simulink model "ikine_test"  (R2019b)
settings: Solver=ode45  StartTime=0.0  StopTime=10.0  RelTol=1e-3  EnableMultiTasking=on
values from neighbouring files (symbols this model uses):
  bL = 22    [runfirst.m]
  bWb = 15.5    [runfirst.m]
  bWs = 13.5    [runfirst.m]
  d1 = 0    [runfirst.m]
  d2 = 0    [runfirst.m]
  L1 = 3.4    [runfirst.m]
  L2 = 9.5    [runfirst.m]
  L3 = 14.2    [runfirst.m]
settings Model: Creator=340DANILOV  LastModifiedBy=root
settings DataIOCC: LimitDataPoints=on  SaveFormat=Array  ReturnWorkspaceOutputs=off
settings OptimizationCC: LifeSpan=inf
settings DebuggingCC: SFUnexpectedBacktrackingDiag=warning  SFNoUnconditionalDefaultTransitionDiag=warning  SFExecutionAtInitializationDiag=none  UnderSpecifiedDimensionMsg=warning  ArithmeticOperatorsInVariantConditions=warning
settings HardwareCC: ProdBitPerPointer=32  ProdBitPerSizeT=32  ProdBitPerPtrDiffT=32  ProdLargestAtomicFloat=None  ProdIntDivRoundTo=Undefined  ProdEndianess=Unspecified  ProdWordSize=32  ProdHWDeviceType=32-bit Generic
settings ModelReferenceCC: PropagateSignalLabelsOutOfModel=off
settings SFSimCC: SimUseLocalCustomCode=off  CustomCodeUndefinedFunction=UseInterfaceOnly
settings RTWCC: RTWUseLocalCustomCode=off
settings CodeAppCC: StateflowObjectComments=on
settings GRTTargetCC: TargetLangStandard=C89/C90 (ANSI)  GeneratePreprocessorConditionals=Disable all
settings ConfigComp: CovMetricSettings=dw  CovHtmlReporting=on  CovSaveCumulativeToWorkspaceVar=on  CovSaveSingleToWorkspaceVar=on  CovExternalEMLEnable=off

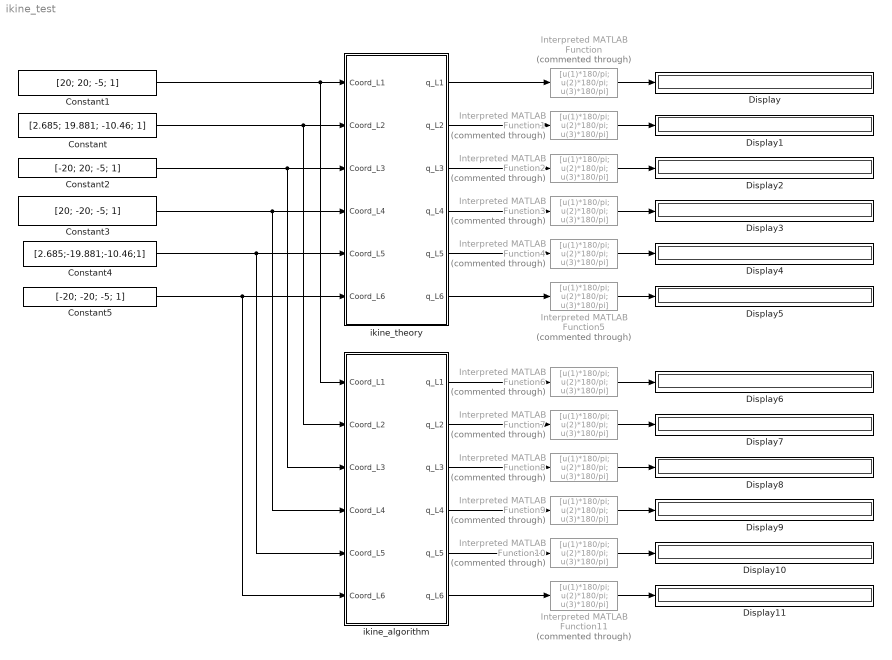
== system ikine_test ==
  Constant : Constant  Value=[2.685; 19.881; -10.46; 1]  VectorParams1D=off
  Constant1 : Constant  Value=[20; 20; -5; 1]  VectorParams1D=off
  Constant2 : Constant  Value=[-20; 20; -5; 1]  VectorParams1D=off
  Constant3 : Constant  Value=[20; -20; -5; 1]  VectorParams1D=off
  Constant4 : Constant  Value=[2.685;-19.881;-10.46;1]  VectorParams1D=off
  Constant5 : Constant  Value=[-20; -20; -5; 1]  VectorParams1D=off
  Display{,1..11} (12 alike) : Display
  Interpreted MATLAB Function{,1..11} (12 alike) : MATLABFcn  Commented=through  MATLABFcn=[u(1)*180/pi; u(2)*180/pi; u(3)*180/pi]
  ikine_algorithm : Subsystem
  ikine_theory : Subsystem
  wires:
  Constant/1 -> ikine_algorithm/2(Coord_L2), ikine_theory/2(Coord_L2)
  Constant1/1 -> ikine_algorithm/1(Coord_L1), ikine_theory/1(Coord_L1)
  Constant2/1 -> ikine_algorithm/3(Coord_L3), ikine_theory/3(Coord_L3)
  Constant3/1 -> ikine_algorithm/4(Coord_L4), ikine_theory/4(Coord_L4)
  Constant4/1 -> ikine_algorithm/5(Coord_L5), ikine_theory/5(Coord_L5)
  Constant5/1 -> ikine_algorithm/6(Coord_L6), ikine_theory/6(Coord_L6)
  Interpreted MATLAB Function/1 -> Display/1
  ikine_theory/1(q_L1) -> Interpreted MATLAB Function/1
  ikine_theory/2(q_L2) -> Interpreted MATLAB Function1/1
  Interpreted MATLAB Function1/1 -> Display1/1
  ikine_theory/3(q_L3) -> Interpreted MATLAB Function2/1
  Interpreted MATLAB Function2/1 -> Display2/1
  ikine_theory/4(q_L4) -> Interpreted MATLAB Function3/1
  Interpreted MATLAB Function3/1 -> Display3/1
  ikine_theory/5(q_L5) -> Interpreted MATLAB Function4/1
  Interpreted MATLAB Function4/1 -> Display4/1
  ikine_theory/6(q_L6) -> Interpreted MATLAB Function5/1
  Interpreted MATLAB Function5/1 -> Display5/1
  ikine_algorithm/1(q_L1) -> Interpreted MATLAB Function6/1
  Interpreted MATLAB Function6/1 -> Display6/1
  ikine_algorithm/2(q_L2) -> Interpreted MATLAB Function7/1
  Interpreted MATLAB Function7/1 -> Display7/1
  ikine_algorithm/3(q_L3) -> Interpreted MATLAB Function8/1
  Interpreted MATLAB Function8/1 -> Display8/1
  ikine_algorithm/4(q_L4) -> Interpreted MATLAB Function9/1
  Interpreted MATLAB Function9/1 -> Display9/1
  ikine_algorithm/5(q_L5) -> Interpreted MATLAB Function10/1
  Interpreted MATLAB Function10/1 -> Display10/1
  ikine_algorithm/6(q_L6) -> Interpreted MATLAB Function11/1
  Interpreted MATLAB Function11/1 -> Display11/1

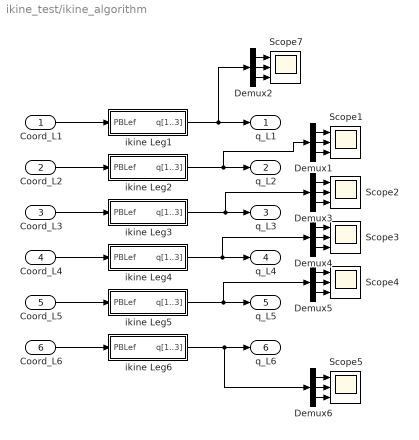
== system ikine_test/ikine_algorithm ==
  Coord_L1 : Inport
  Coord_L2 : Inport  Port=2
  Coord_L3 : Inport  Port=3
  Coord_L4 : Inport  Port=4
  Coord_L5 : Inport  Port=5
  Coord_L6 : Inport  Port=6
  Demux{1..6} (6 alike) : Demux  Outputs=3
  Scope{1..5,7} (6 alike) : Scope  NumInputPorts=3
  ikine Leg1 : Subsystem
  ikine Leg2 : Subsystem
  ikine Leg3 : Subsystem
  ikine Leg4 : Subsystem
  ikine Leg5 : Subsystem
  ikine Leg6 : Subsystem
  q_L1 : Outport  VectorParamsAs1DForOutWhenUnconnected=off
  q_L2 : Outport  Port=2  VectorParamsAs1DForOutWhenUnconnected=off
  q_L3 : Outport  Port=3  VectorParamsAs1DForOutWhenUnconnected=off
  q_L4 : Outport  Port=4  VectorParamsAs1DForOutWhenUnconnected=off
  q_L5 : Outport  Port=5  VectorParamsAs1DForOutWhenUnconnected=off
  q_L6 : Outport  Port=6  VectorParamsAs1DForOutWhenUnconnected=off
  wires:
  Demux6/1 -> Scope5/1
  Demux6/2 -> Scope5/2
  Demux6/3 -> Scope5/3
  Demux5/1 -> Scope4/1
  Demux5/2 -> Scope4/2
  Demux5/3 -> Scope4/3
  Demux4/1 -> Scope3/1
  Demux4/2 -> Scope3/2
  Demux4/3 -> Scope3/3
  Demux3/1 -> Scope2/1
  Demux3/2 -> Scope2/2
  Demux3/3 -> Scope2/3
  Demux1/1 -> Scope1/1
  Demux1/2 -> Scope1/2
  Demux1/3 -> Scope1/3
  Demux2/1 -> Scope7/1
  Demux2/2 -> Scope7/2
  Demux2/3 -> Scope7/3
  Coord_L6/1 -> ikine Leg6/1(PBLef)
  Coord_L5/1 -> ikine Leg5/1(PBLef)
  Coord_L4/1 -> ikine Leg4/1(PBLef)
  Coord_L3/1 -> ikine Leg3/1(PBLef)
  Coord_L2/1 -> ikine Leg2/1(PBLef)
  Coord_L1/1 -> ikine Leg1/1(PBLef)
  ikine Leg6/1(q[1..3]) -> q_L6/1, Demux6/1
  ikine Leg5/1(q[1..3]) -> q_L5/1, Demux5/1
  ikine Leg4/1(q[1..3]) -> q_L4/1, Demux4/1
  ikine Leg3/1(q[1..3]) -> q_L3/1, Demux3/1
  ikine Leg2/1(q[1..3]) -> q_L2/1, Demux1/1
  ikine Leg1/1(q[1..3]) -> q_L1/1, Demux2/1

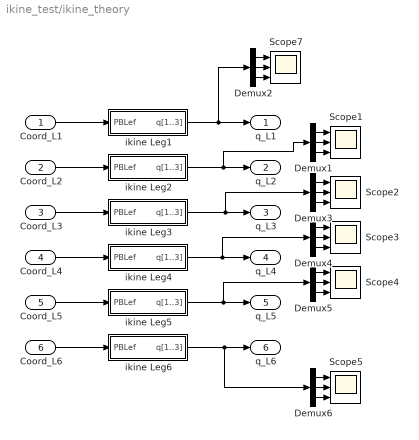
== system ikine_test/ikine_theory ==
  Coord_L1 : Inport
  Coord_L2 : Inport  Port=2
  Coord_L3 : Inport  Port=3
  Coord_L4 : Inport  Port=4
  Coord_L5 : Inport  Port=5
  Coord_L6 : Inport  Port=6
  Demux{1..6} (6 alike) : Demux  Outputs=3
  Scope{1..5,7} (6 alike) : Scope  NumInputPorts=3
  ikine Leg1 : Subsystem
  ikine Leg2 : Subsystem
  ikine Leg3 : Subsystem
  ikine Leg4 : Subsystem
  ikine Leg5 : Subsystem
  ikine Leg6 : Subsystem
  q_L1 : Outport  VectorParamsAs1DForOutWhenUnconnected=off
  q_L2 : Outport  Port=2  VectorParamsAs1DForOutWhenUnconnected=off
  q_L3 : Outport  Port=3  VectorParamsAs1DForOutWhenUnconnected=off
  q_L4 : Outport  Port=4  VectorParamsAs1DForOutWhenUnconnected=off
  q_L5 : Outport  Port=5  VectorParamsAs1DForOutWhenUnconnected=off
  q_L6 : Outport  Port=6  VectorParamsAs1DForOutWhenUnconnected=off
  wires:
  Demux6/1 -> Scope5/1
  Demux6/2 -> Scope5/2
  Demux6/3 -> Scope5/3
  Demux5/1 -> Scope4/1
  Demux5/2 -> Scope4/2
  Demux5/3 -> Scope4/3
  Demux4/1 -> Scope3/1
  Demux4/2 -> Scope3/2
  Demux4/3 -> Scope3/3
  Demux3/1 -> Scope2/1
  Demux3/2 -> Scope2/2
  Demux3/3 -> Scope2/3
  Demux1/1 -> Scope1/1
  Demux1/2 -> Scope1/2
  Demux1/3 -> Scope1/3
  Demux2/1 -> Scope7/1
  Demux2/2 -> Scope7/2
  Demux2/3 -> Scope7/3
  Coord_L6/1 -> ikine Leg6/1(PBLef)
  Coord_L5/1 -> ikine Leg5/1(PBLef)
  Coord_L4/1 -> ikine Leg4/1(PBLef)
  Coord_L3/1 -> ikine Leg3/1(PBLef)
  Coord_L2/1 -> ikine Leg2/1(PBLef)
  Coord_L1/1 -> ikine Leg1/1(PBLef)
  ikine Leg6/1(q[1..3]) -> q_L6/1, Demux6/1
  ikine Leg5/1(q[1..3]) -> q_L5/1, Demux5/1
  ikine Leg4/1(q[1..3]) -> q_L4/1, Demux4/1
  ikine Leg3/1(q[1..3]) -> q_L3/1, Demux3/1
  ikine Leg2/1(q[1..3]) -> q_L2/1, Demux1/1
  ikine Leg1/1(q[1..3]) -> q_L1/1, Demux2/1

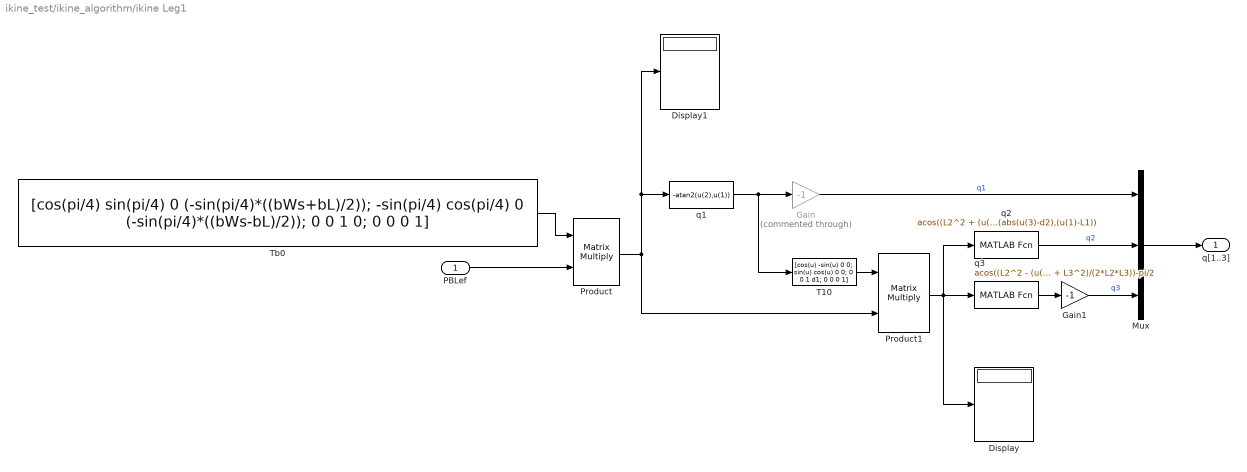
== system ikine_test/ikine_algorithm/ikine Leg1 ==
  PBLef : Inport
  Display : Display
  Display1 : Display
  Gain : Gain  Commented=through  Gain=-1
  Gain1 : Gain  Gain=-1
  Mux : Mux  Inputs=3
  Product : Product  Multiplication=Matrix(*)
  Product1 : Product  Multiplication=Matrix(*)
  T10 : MATLABFcn  MATLABFcn=[cos(u) -sin(u) 0 0; sin(u) cos(u) 0 0; 0 0 1 d1; 0 0 0 1]  OutputDimensions=[4;4]  Output1D=off
  Tb0 : Constant  Value=[cos(pi/4) sin(pi/4) 0 (-sin(pi/4)*((bWs+bL)/2)); -sin(pi/4) cos(pi/4) 0 (-sin(pi/4)*((bWs-bL)/2)); 0 0 1 0; 0 0 0 1]  VectorParams1D=off
  q1 : MATLABFcn  MATLABFcn=-atan2(u(2),u(1))
  q2 : MATLABFcn  MATLABFcn=acos((L2^2 + (u(1)-L1)^2 + (u(3)-d2)^2 - L3^2)/(2*L2*sqrt((u(1)-L1)^2+(u(3)-d2)^2)))-atan2(abs(u(3)-d2),(u(1)-L1))
  q3 : MATLABFcn  MATLABFcn=acos((L2^2 - (u(1)-L1)^2 - (u(3)-d2)^2 + L3^2)/(2*L2*L3))-pi/2
  q[1..3] : Outport  VectorParamsAs1DForOutWhenUnconnected=off
  wires:
  Gain1/1 -> Mux/3  "q3"
  Tb0/1 -> Product/1
  PBLef/1 -> Product/2
  Product/1 -> Display1/1, q1/1, Product1/2
  q1/1 -> T10/1, Gain/1
  q2/1 -> Mux/2  "q2"
  T10/1 -> Product1/1
  Product1/1 -> Display/1, q3/1, q2/1
  q3/1 -> Gain1/1
  Gain/1 -> Mux/1  "q1"
  Mux/1 -> q[1..3]/1

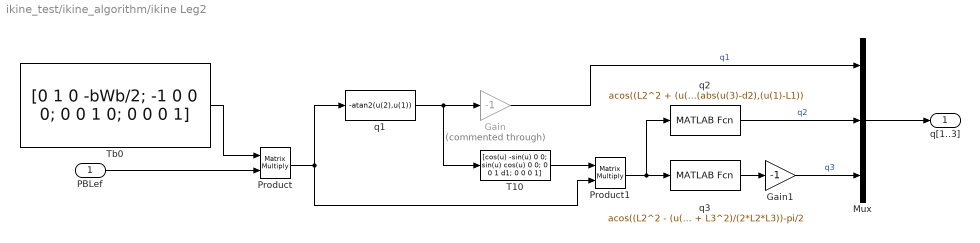
== system ikine_test/ikine_algorithm/ikine Leg2 ==
  PBLef : Inport
  Gain : Gain  Commented=through  Gain=-1
  Gain1 : Gain  Gain=-1
  Mux : Mux  Inputs=3
  Product : Product  Multiplication=Matrix(*)
  Product1 : Product  Multiplication=Matrix(*)
  T10 : MATLABFcn  MATLABFcn=[cos(u) -sin(u) 0 0; sin(u) cos(u) 0 0; 0 0 1 d1; 0 0 0 1]  OutputDimensions=[4;4]  Output1D=off
  Tb0 : Constant  Value=[0 1 0 -bWb/2; -1 0 0 0; 0 0 1 0; 0 0 0 1]  VectorParams1D=off
  q1 : MATLABFcn  MATLABFcn=-atan2(u(2),u(1))
  q2 : MATLABFcn  MATLABFcn=acos((L2^2 + (u(1)-L1)^2 + (u(3)-d2)^2 - L3^2)/(2*L2*sqrt((u(1)-L1)^2+(u(3)-d2)^2)))-atan2(abs(u(3)-d2),(u(1)-L1))
  q3 : MATLABFcn  MATLABFcn=acos((L2^2 - (u(1)-L1)^2 - (u(3)-d2)^2 + L3^2)/(2*L2*L3))-pi/2
  q[1..3] : Outport  VectorParamsAs1DForOutWhenUnconnected=off
  wires:
  Gain1/1 -> Mux/3  "q3"
  Tb0/1 -> Product/1
  PBLef/1 -> Product/2
  Product/1 -> q1/1, Product1/2
  q1/1 -> T10/1, Gain/1
  q2/1 -> Mux/2  "q2"
  T10/1 -> Product1/1
  Product1/1 -> q3/1, q2/1
  q3/1 -> Gain1/1
  Gain/1 -> Mux/1  "q1"
  Mux/1 -> q[1..3]/1

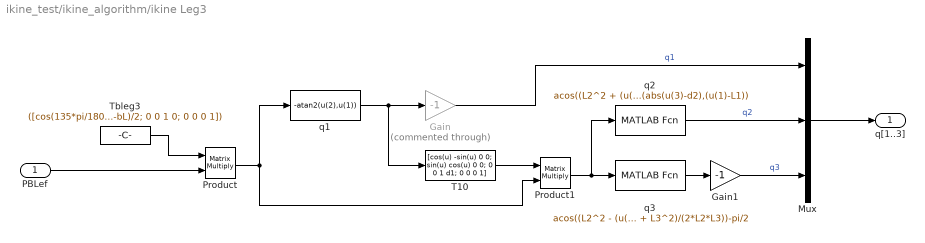
== system ikine_test/ikine_algorithm/ikine Leg3 ==
  PBLef : Inport
  Gain : Gain  Commented=through  Gain=-1
  Gain1 : Gain  Gain=-1
  Mux : Mux  Inputs=3
  Product : Product  Multiplication=Matrix(*)
  Product1 : Product  Multiplication=Matrix(*)
  T10 : MATLABFcn  MATLABFcn=[cos(u) -sin(u) 0 0; sin(u) cos(u) 0 0; 0 0 1 d1; 0 0 0 1]  OutputDimensions=[4;4]  Output1D=off
  Tbleg3 : Constant  Value=([cos(135*pi/180) sin(135*pi/180) 0 -sin(pi/4)*(bWs+bL)/2; sin(-135*pi/180) cos(135*pi/180) 0 sin(pi/4)*(bWs-bL)/2; 0 0 1 0; 0 0 0 1])  VectorParams1D=off
  q1 : MATLABFcn  MATLABFcn=-atan2(u(2),u(1))
  q2 : MATLABFcn  MATLABFcn=acos((L2^2 + (u(1)-L1)^2 + (u(3)-d2)^2 - L3^2)/(2*L2*sqrt((u(1)-L1)^2+(u(3)-d2)^2)))-atan2(abs(u(3)-d2),(u(1)-L1))
  q3 : MATLABFcn  MATLABFcn=acos((L2^2 - (u(1)-L1)^2 - (u(3)-d2)^2 + L3^2)/(2*L2*L3))-pi/2
  q[1..3] : Outport  VectorParamsAs1DForOutWhenUnconnected=off
  wires:
  Mux/1 -> q[1..3]/1
  Gain/1 -> Mux/1  "q1"
  q3/1 -> Gain1/1
  Product1/1 -> q2/1, q3/1
  T10/1 -> Product1/1
  q2/1 -> Mux/2  "q2"
  q1/1 -> T10/1, Gain/1
  Product/1 -> Product1/2, q1/1
  PBLef/1 -> Product/2
  Tbleg3/1 -> Product/1
  Gain1/1 -> Mux/3  "q3"

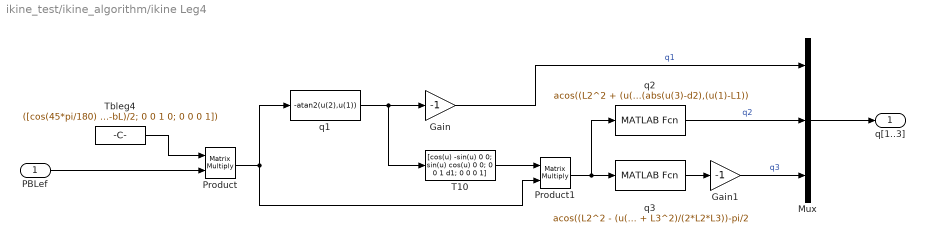
== system ikine_test/ikine_algorithm/ikine Leg4 ==
  PBLef : Inport
  Gain : Gain  Gain=-1
  Gain1 : Gain  Gain=-1
  Mux : Mux  Inputs=3
  Product : Product  Multiplication=Matrix(*)
  Product1 : Product  Multiplication=Matrix(*)
  T10 : MATLABFcn  MATLABFcn=[cos(u) -sin(u) 0 0; sin(u) cos(u) 0 0; 0 0 1 d1; 0 0 0 1]  OutputDimensions=[4;4]  Output1D=off
  Tbleg4 : Constant  Value=([cos(45*pi/180) -sin(45*pi/180) 0 -sin(pi/4)*(bWs+bL)/2; sin(45*pi/180) cos(45*pi/180) 0 sin(pi/4)*(bWs-bL)/2; 0 0 1 0; 0 0 0 1])  VectorParams1D=off
  q1 : MATLABFcn  MATLABFcn=-atan2(u(2),u(1))
  q2 : MATLABFcn  MATLABFcn=acos((L2^2 + (u(1)-L1)^2 + (u(3)-d2)^2 - L3^2)/(2*L2*sqrt((u(1)-L1)^2+(u(3)-d2)^2)))-atan2(abs(u(3)-d2),(u(1)-L1))
  q3 : MATLABFcn  MATLABFcn=acos((L2^2 - (u(1)-L1)^2 - (u(3)-d2)^2 + L3^2)/(2*L2*L3))-pi/2
  q[1..3] : Outport  VectorParamsAs1DForOutWhenUnconnected=off
  wires:
  Gain1/1 -> Mux/3  "q3"
  Tbleg4/1 -> Product/1
  PBLef/1 -> Product/2
  Product/1 -> q1/1, Product1/2
  q1/1 -> T10/1, Gain/1
  q2/1 -> Mux/2  "q2"
  T10/1 -> Product1/1
  Product1/1 -> q3/1, q2/1
  q3/1 -> Gain1/1
  Gain/1 -> Mux/1  "q1"
  Mux/1 -> q[1..3]/1

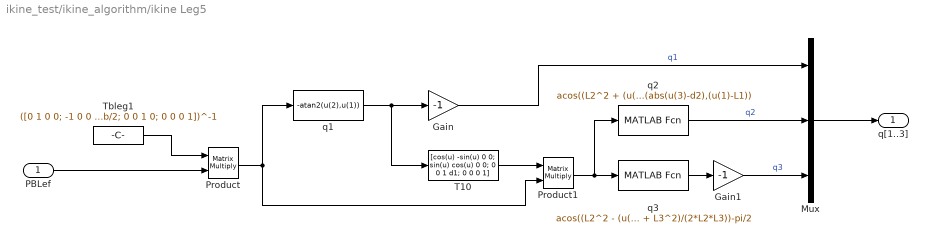
== system ikine_test/ikine_algorithm/ikine Leg5 ==
  PBLef : Inport
  Gain : Gain  Gain=-1
  Gain1 : Gain  Gain=-1
  Mux : Mux  Inputs=3
  Product : Product  Multiplication=Matrix(*)
  Product1 : Product  Multiplication=Matrix(*)
  T10 : MATLABFcn  MATLABFcn=[cos(u) -sin(u) 0 0; sin(u) cos(u) 0 0; 0 0 1 d1; 0 0 0 1]  OutputDimensions=[4;4]  Output1D=off
  Tbleg1 : Constant  Value=([0 1 0 0; -1 0 0 -bWb/2; 0 0 1 0; 0 0 0 1])^-1  VectorParams1D=off
  q1 : MATLABFcn  MATLABFcn=-atan2(u(2),u(1))
  q2 : MATLABFcn  MATLABFcn=acos((L2^2 + (u(1)-L1)^2 + (u(3)-d2)^2 - L3^2)/(2*L2*sqrt((u(1)-L1)^2+(u(3)-d2)^2)))-atan2(abs(u(3)-d2),(u(1)-L1))
  q3 : MATLABFcn  MATLABFcn=acos((L2^2 - (u(1)-L1)^2 - (u(3)-d2)^2 + L3^2)/(2*L2*L3))-pi/2
  q[1..3] : Outport  VectorParamsAs1DForOutWhenUnconnected=off
  wires:
  Mux/1 -> q[1..3]/1
  Gain/1 -> Mux/1  "q1"
  q3/1 -> Gain1/1
  Product1/1 -> q2/1, q3/1
  T10/1 -> Product1/1
  q2/1 -> Mux/2  "q2"
  q1/1 -> T10/1, Gain/1
  Product/1 -> Product1/2, q1/1
  PBLef/1 -> Product/2
  Tbleg1/1 -> Product/1
  Gain1/1 -> Mux/3  "q3"

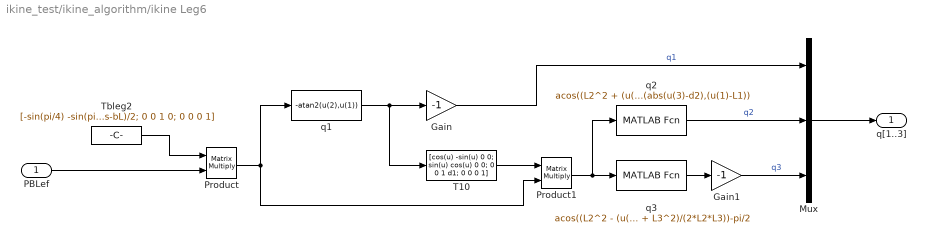
== system ikine_test/ikine_algorithm/ikine Leg6 ==
  PBLef : Inport
  Gain : Gain  Gain=-1
  Gain1 : Gain  Gain=-1
  Mux : Mux  Inputs=3
  Product : Product  Multiplication=Matrix(*)
  Product1 : Product  Multiplication=Matrix(*)
  T10 : MATLABFcn  MATLABFcn=[cos(u) -sin(u) 0 0; sin(u) cos(u) 0 0; 0 0 1 d1; 0 0 0 1]  OutputDimensions=[4;4]  Output1D=off
  Tbleg2 : Constant  Value=[-sin(pi/4) -sin(pi/4) 0 -sin(pi/4)*(bWs+bL)/2; sin(pi/4) -sin(pi/4) 0 -sin(pi/4)*(bWs-bL)/2; 0 0 1 0; 0 0 0 1]  VectorParams1D=off
  q1 : MATLABFcn  MATLABFcn=-atan2(u(2),u(1))
  q2 : MATLABFcn  MATLABFcn=acos((L2^2 + (u(1)-L1)^2 + (u(3)-d2)^2 - L3^2)/(2*L2*sqrt((u(1)-L1)^2+(u(3)-d2)^2)))-atan2(abs(u(3)-d2),(u(1)-L1))
  q3 : MATLABFcn  MATLABFcn=acos((L2^2 - (u(1)-L1)^2 - (u(3)-d2)^2 + L3^2)/(2*L2*L3))-pi/2
  q[1..3] : Outport  VectorParamsAs1DForOutWhenUnconnected=off
  wires:
  Mux/1 -> q[1..3]/1
  Gain/1 -> Mux/1  "q1"
  q3/1 -> Gain1/1
  Product1/1 -> q2/1, q3/1
  T10/1 -> Product1/1
  q2/1 -> Mux/2  "q2"
  q1/1 -> T10/1, Gain/1
  Product/1 -> Product1/2, q1/1
  PBLef/1 -> Product/2
  Tbleg2/1 -> Product/1
  Gain1/1 -> Mux/3  "q3"

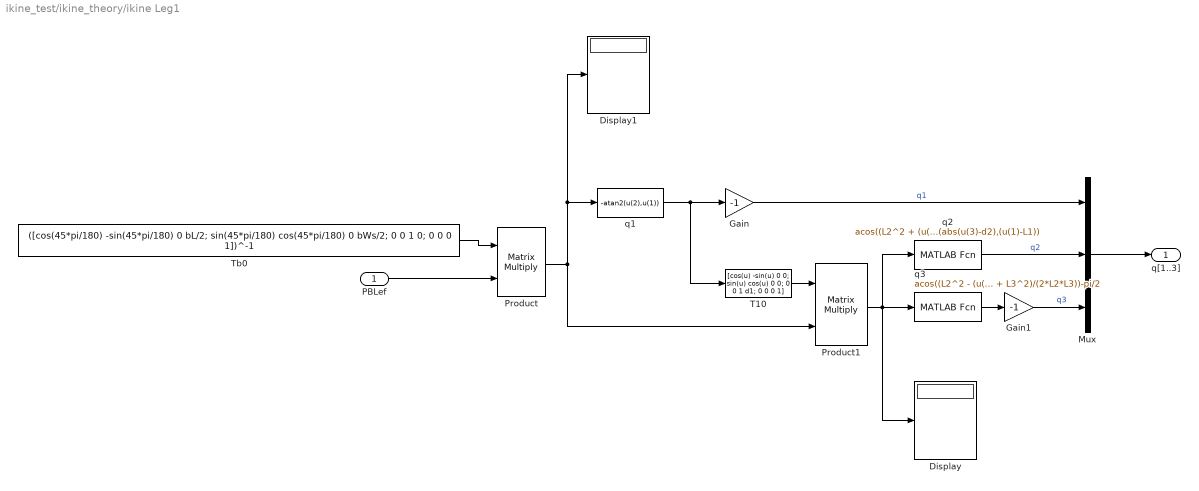
== system ikine_test/ikine_theory/ikine Leg1 ==
  PBLef : Inport
  Display : Display
  Display1 : Display
  Gain : Gain  Gain=-1
  Gain1 : Gain  Gain=-1
  Mux : Mux  Inputs=3
  Product : Product  Multiplication=Matrix(*)
  Product1 : Product  Multiplication=Matrix(*)
  T10 : MATLABFcn  MATLABFcn=[cos(u) -sin(u) 0 0; sin(u) cos(u) 0 0; 0 0 1 d1; 0 0 0 1]  Output1D=off
  Tb0 : Constant  Value=([cos(45*pi/180) -sin(45*pi/180) 0 bL/2; sin(45*pi/180) cos(45*pi/180) 0 bWs/2; 0 0 1 0; 0 0 0 1])^-1  VectorParams1D=off
  q1 : MATLABFcn  MATLABFcn=-atan2(u(2),u(1))
  q2 : MATLABFcn  MATLABFcn=acos((L2^2 + (u(1)-L1)^2 + (u(3)-d2)^2 - L3^2)/(2*L2*sqrt((u(1)-L1)^2+(u(3)-d2)^2)))-atan2(abs(u(3)-d2),(u(1)-L1))
  q3 : MATLABFcn  MATLABFcn=acos((L2^2 - (u(1)-L1)^2 - (u(3)-d2)^2 + L3^2)/(2*L2*L3))-pi/2
  q[1..3] : Outport  VectorParamsAs1DForOutWhenUnconnected=off
  wires:
  Gain1/1 -> Mux/3  "q3"
  Tb0/1 -> Product/1
  PBLef/1 -> Product/2
  Product/1 -> Display1/1, q1/1, Product1/2
  q1/1 -> T10/1, Gain/1
  q2/1 -> Mux/2  "q2"
  T10/1 -> Product1/1
  Product1/1 -> Display/1, q3/1, q2/1
  q3/1 -> Gain1/1
  Gain/1 -> Mux/1  "q1"
  Mux/1 -> q[1..3]/1

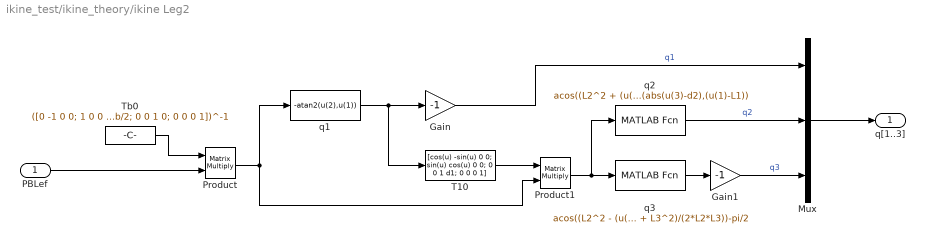
== system ikine_test/ikine_theory/ikine Leg2 ==
  PBLef : Inport
  Gain : Gain  Gain=-1
  Gain1 : Gain  Gain=-1
  Mux : Mux  Inputs=3
  Product : Product  Multiplication=Matrix(*)
  Product1 : Product  Multiplication=Matrix(*)
  T10 : MATLABFcn  MATLABFcn=[cos(u) -sin(u) 0 0; sin(u) cos(u) 0 0; 0 0 1 d1; 0 0 0 1]  OutputDimensions=[4;4]  Output1D=off
  Tb0 : Constant  Value=([0 -1 0 0; 1 0 0 bWb/2; 0 0 1 0; 0 0 0 1])^-1  VectorParams1D=off
  q1 : MATLABFcn  MATLABFcn=-atan2(u(2),u(1))
  q2 : MATLABFcn  MATLABFcn=acos((L2^2 + (u(1)-L1)^2 + (u(3)-d2)^2 - L3^2)/(2*L2*sqrt((u(1)-L1)^2+(u(3)-d2)^2)))-atan2(abs(u(3)-d2),(u(1)-L1))
  q3 : MATLABFcn  MATLABFcn=acos((L2^2 - (u(1)-L1)^2 - (u(3)-d2)^2 + L3^2)/(2*L2*L3))-pi/2
  q[1..3] : Outport  VectorParamsAs1DForOutWhenUnconnected=off
  wires:
  Gain1/1 -> Mux/3  "q3"
  Tb0/1 -> Product/1
  PBLef/1 -> Product/2
  Product/1 -> q1/1, Product1/2
  q1/1 -> T10/1, Gain/1
  q2/1 -> Mux/2  "q2"
  T10/1 -> Product1/1
  Product1/1 -> q3/1, q2/1
  q3/1 -> Gain1/1
  Gain/1 -> Mux/1  "q1"
  Mux/1 -> q[1..3]/1

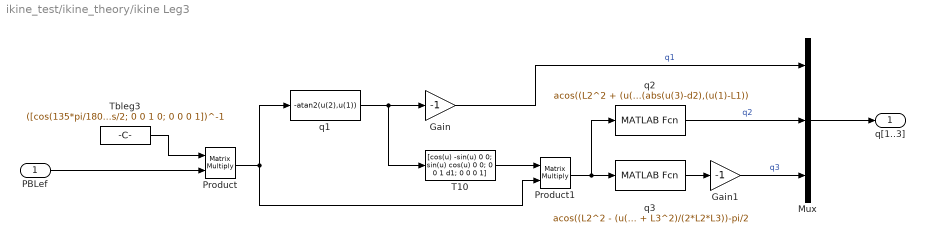
== system ikine_test/ikine_theory/ikine Leg3 ==
  PBLef : Inport
  Gain : Gain  Gain=-1
  Gain1 : Gain  Gain=-1
  Mux : Mux  Inputs=3
  Product : Product  Multiplication=Matrix(*)
  Product1 : Product  Multiplication=Matrix(*)
  T10 : MATLABFcn  MATLABFcn=[cos(u) -sin(u) 0 0; sin(u) cos(u) 0 0; 0 0 1 d1; 0 0 0 1]  OutputDimensions=[4;4]  Output1D=off
  Tbleg3 : Constant  Value=([cos(135*pi/180) -sin(135*pi/180) 0 -bL/2; sin(135*pi/180) cos(135*pi/180) 0 bWs/2; 0 0 1 0; 0 0 0 1])^-1  VectorParams1D=off
  q1 : MATLABFcn  MATLABFcn=-atan2(u(2),u(1))
  q2 : MATLABFcn  MATLABFcn=acos((L2^2 + (u(1)-L1)^2 + (u(3)-d2)^2 - L3^2)/(2*L2*sqrt((u(1)-L1)^2+(u(3)-d2)^2)))-atan2(abs(u(3)-d2),(u(1)-L1))
  q3 : MATLABFcn  MATLABFcn=acos((L2^2 - (u(1)-L1)^2 - (u(3)-d2)^2 + L3^2)/(2*L2*L3))-pi/2
  q[1..3] : Outport  VectorParamsAs1DForOutWhenUnconnected=off
  wires:
  Mux/1 -> q[1..3]/1
  Gain/1 -> Mux/1  "q1"
  q3/1 -> Gain1/1
  Product1/1 -> q2/1, q3/1
  T10/1 -> Product1/1
  q2/1 -> Mux/2  "q2"
  q1/1 -> T10/1, Gain/1
  Product/1 -> Product1/2, q1/1
  PBLef/1 -> Product/2
  Tbleg3/1 -> Product/1
  Gain1/1 -> Mux/3  "q3"

== system ikine_test/ikine_theory/ikine Leg4 ==
  PBLef : Inport
  Gain : Gain  Gain=-1
  Gain1 : Gain  Gain=-1
  Mux : Mux  Inputs=3
  Product : Product  Multiplication=Matrix(*)
  Product1 : Product  Multiplication=Matrix(*)
  T10 : MATLABFcn  MATLABFcn=[cos(u) -sin(u) 0 0; sin(u) cos(u) 0 0; 0 0 1 d1; 0 0 0 1]  OutputDimensions=[4;4]  Output1D=off
  Tbleg4 : Constant  Value=([cos(-45*pi/180) -sin(-45*pi/180) 0 bL/2; sin(-45*pi/180) cos(-45*pi/180) 0 -bWs/2; 0 0 1 0; 0 0 0 1])^-1  VectorParams1D=off
  q1 : MATLABFcn  MATLABFcn=-atan2(u(2),u(1))
  q2 : MATLABFcn  MATLABFcn=acos((L2^2 + (u(1)-L1)^2 + (u(3)-d2)^2 - L3^2)/(2*L2*sqrt((u(1)-L1)^2+(u(3)-d2)^2)))-atan2(abs(u(3)-d2),(u(1)-L1))
  q3 : MATLABFcn  MATLABFcn=acos((L2^2 - (u(1)-L1)^2 - (u(3)-d2)^2 + L3^2)/(2*L2*L3))-pi/2
  q[1..3] : Outport  VectorParamsAs1DForOutWhenUnconnected=off
  wires:
  Gain1/1 -> Mux/3  "q3"
  Tbleg4/1 -> Product/1
  PBLef/1 -> Product/2
  Product/1 -> q1/1, Product1/2
  q1/1 -> T10/1, Gain/1
  q2/1 -> Mux/2  "q2"
  T10/1 -> Product1/1
  Product1/1 -> q3/1, q2/1
  q3/1 -> Gain1/1
  Gain/1 -> Mux/1  "q1"
  Mux/1 -> q[1..3]/1

== system ikine_test/ikine_theory/ikine Leg5 ==
  PBLef : Inport
  Gain : Gain  Gain=-1
  Gain1 : Gain  Gain=-1
  Mux : Mux  Inputs=3
  Product : Product  Multiplication=Matrix(*)
  Product1 : Product  Multiplication=Matrix(*)
  T10 : MATLABFcn  MATLABFcn=[cos(u) -sin(u) 0 0; sin(u) cos(u) 0 0; 0 0 1 d1; 0 0 0 1]  OutputDimensions=[4;4]  Output1D=off
  Tbleg1 : Constant  Value=([0 1 0 0; -1 0 0 -bWb/2; 0 0 1 0; 0 0 0 1])^-1  VectorParams1D=off
  q1 : MATLABFcn  MATLABFcn=-atan2(u(2),u(1))
  q2 : MATLABFcn  MATLABFcn=acos((L2^2 + (u(1)-L1)^2 + (u(3)-d2)^2 - L3^2)/(2*L2*sqrt((u(1)-L1)^2+(u(3)-d2)^2)))-atan2(abs(u(3)-d2),(u(1)-L1))
  q3 : MATLABFcn  MATLABFcn=acos((L2^2 - (u(1)-L1)^2 - (u(3)-d2)^2 + L3^2)/(2*L2*L3))-pi/2
  q[1..3] : Outport  VectorParamsAs1DForOutWhenUnconnected=off
  wires:
  Mux/1 -> q[1..3]/1
  Gain/1 -> Mux/1  "q1"
  q3/1 -> Gain1/1
  Product1/1 -> q2/1, q3/1
  T10/1 -> Product1/1
  q2/1 -> Mux/2  "q2"
  q1/1 -> T10/1, Gain/1
  Product/1 -> Product1/2, q1/1
  PBLef/1 -> Product/2
  Tbleg1/1 -> Product/1
  Gain1/1 -> Mux/3  "q3"

== system ikine_test/ikine_theory/ikine Leg6 ==
  PBLef : Inport
  Gain : Gain  Gain=-1
  Gain1 : Gain  Gain=-1
  Mux : Mux  Inputs=3
  Product : Product  Multiplication=Matrix(*)
  Product1 : Product  Multiplication=Matrix(*)
  T10 : MATLABFcn  MATLABFcn=[cos(u) -sin(u) 0 0; sin(u) cos(u) 0 0; 0 0 1 d1; 0 0 0 1]  OutputDimensions=[4;4]  Output1D=off
  Tbleg2 : Constant  Value=([cos(-135*pi/180) -sin(-135*pi/180) 0 -bL/2; sin(-135*pi/180) cos(-135*pi/180) 0 -bWs/2; 0 0 1 0; 0 0 0 1])^-1  VectorParams1D=off
  q1 : MATLABFcn  MATLABFcn=-atan2(u(2),u(1))
  q2 : MATLABFcn  MATLABFcn=acos((L2^2 + (u(1)-L1)^2 + (u(3)-d2)^2 - L3^2)/(2*L2*sqrt((u(1)-L1)^2+(u(3)-d2)^2)))-atan2(abs(u(3)-d2),(u(1)-L1))
  q3 : MATLABFcn  MATLABFcn=acos((L2^2 - (u(1)-L1)^2 - (u(3)-d2)^2 + L3^2)/(2*L2*L3))-pi/2
  q[1..3] : Outport  VectorParamsAs1DForOutWhenUnconnected=off
  wires:
  Mux/1 -> q[1..3]/1
  Gain/1 -> Mux/1  "q1"
  q3/1 -> Gain1/1
  Product1/1 -> q2/1, q3/1
  T10/1 -> Product1/1
  q2/1 -> Mux/2  "q2"
  q1/1 -> T10/1, Gain/1
  Product/1 -> Product1/2, q1/1
  PBLef/1 -> Product/2
  Tbleg2/1 -> Product/1
  Gain1/1 -> Mux/3  "q3"
